simulink model "ctrl_enhanced"  (R2018b)
settings: Solver=VariableStepAuto  StartTime=0.0  StopTime=10.0  RelTol=1e-3
values from neighbouring files (symbols this model uses):
  T = 0.005    [robot_setup.m]
settings Model: Creator=alberto  LastModifiedBy=alberto

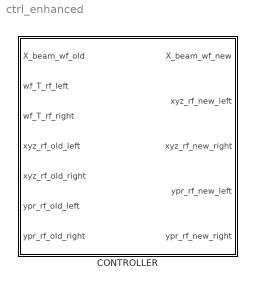
== system ctrl_enhanced ==
  CONTROLLER : Subsystem

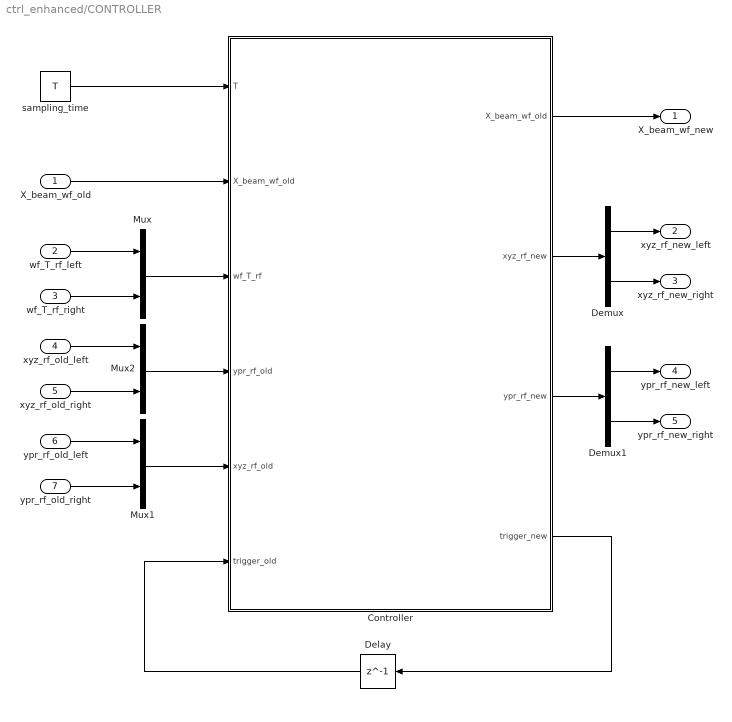
== system ctrl_enhanced/CONTROLLER ==
  X_beam_wf_old : Inport
  wf_T_rf_left : Inport  Port=2
  wf_T_rf_right : Inport  Port=3
  "xyz_rf_old_left " : Inport  Port=4
  xyz_rf_old_right : Inport  Port=5
  ypr_rf_old_left : Inport  Port=6
  ypr_rf_old_right : Inport  Port=7
  Controller : MATLAB Function  TreatAsAtomicUnit=on
  Delay : Delay  DelayLength=1  InitialCondition=zeros(5,1)
  Demux : Demux  Outputs=2
  Demux1 : Demux  Outputs=2
  Mux : Mux  Inputs=2
  Mux1 : Mux  Inputs=2
  Mux2 : Mux  Inputs=2
  sampling_time : Constant  Value=T
  X_beam_wf_new : Outport
  xyz_rf_new_left : Outport  Port=2
  xyz_rf_new_right : Outport  Port=3
  ypr_rf_new_left : Outport  Port=4
  ypr_rf_new_right : Outport  Port=5
  wires:
  Controller/1(X_beam_wf_old) -> X_beam_wf_new/1
  Delay/1 -> Controller/6(trigger_old)
  Controller/4(trigger_new) -> Delay/1
  sampling_time/1 -> Controller/1(T)
  X_beam_wf_old/1 -> Controller/2("X_beam_wf_old ")
  wf_T_rf_left/1 -> Mux/1
  wf_T_rf_right/1 -> Mux/2
  Mux/1 -> Controller/3(wf_T_rf)
  ypr_rf_old_left/1 -> Mux1/1
  ypr_rf_old_right/1 -> Mux1/2
  Mux1/1 -> Controller/5(xyz_rf_old)
  "xyz_rf_old_left "/1 -> Mux2/1
  xyz_rf_old_right/1 -> Mux2/2
  Mux2/1 -> Controller/4(ypr_rf_old)
  Controller/2(xyz_rf_new) -> Demux/1
  Demux/1 -> xyz_rf_new_left/1
  Demux/2 -> xyz_rf_new_right/1
  Controller/3(ypr_rf_new) -> Demux1/1
  Demux1/1 -> ypr_rf_new_left/1
  Demux1/2 -> ypr_rf_new_right/1

== matlab function ctrl_enhanced/CONTROLLER/Controller ==
  data: T input; X_beam_wf_old output; xyz_rf_new output; X_beam_wf_old input; wf_T_rf input; ypr_rf_old input; xyz_rf_old input; trigger_old input; ypr_rf_new output; trigger_new output
function [X_beam_wf_old, xyz_rf_new, ypr_rf_new, trigger_new] = robot_ctrl(T, X_beam_wf_old, wf_T_rf, ypr_rf_old, xyz_rf_old, trigger_old)






end
